simulink subsystem "drone_model"  (R2023a)
settings: Solver=VariableStepAuto  StartTime=0.0  StopTime=10.0  RelTol=1e-3
values from neighbouring files (symbols this model uses):
  G = [kF kF kF kF ... (first row only)    [config.m]
  Ginv = inv(G)    [config.m]
  k_loss = 1.219    [config.m]
  kF = -0.00019205 / 1.225    (= -0.000156775510204)    [config.m]
  kM = 4.90694039e-06 / 1.225    (= 4.00566562449e-06)    [config.m]
undefined symbols (not defined in the file or in its folder): param
libraries: shared6dof x1
settings Model: Creator=timme  LastModifiedBy=timme

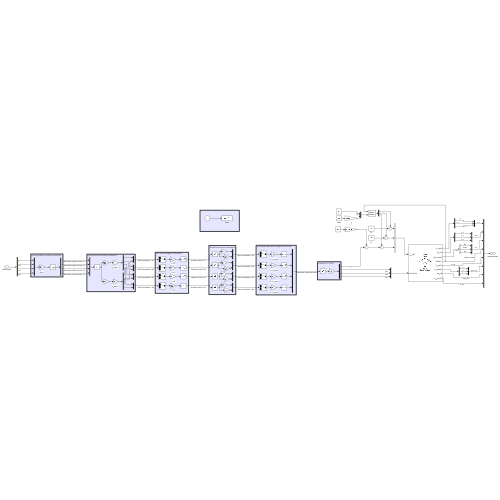
[thumbnail: Simulink's stored preview of the top-level diagram]
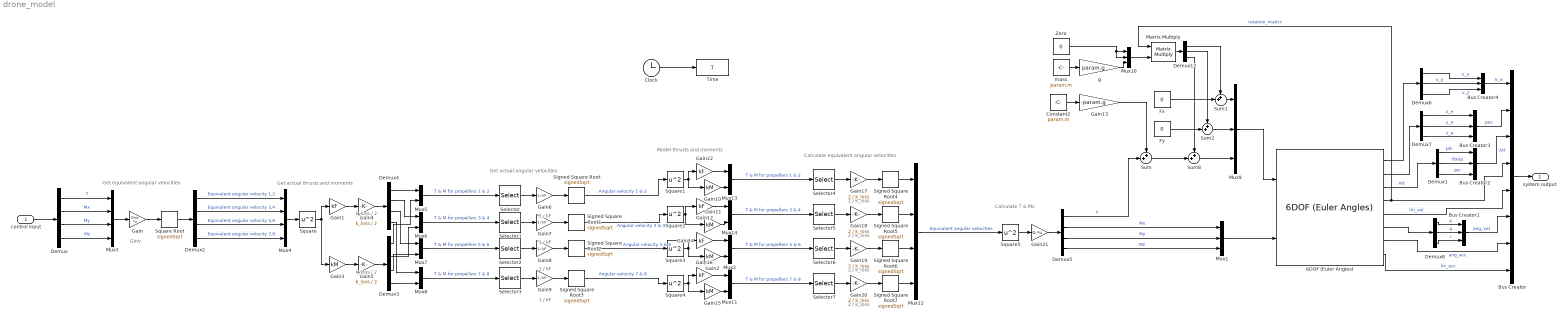
== system drone_model ==
  note: 1 / kF
  note: Calculate equivalent angular velocities
  note: Model thrusts and moments
  note: k_loss / 2
  note: Calculate T & Ms
  note: 2 / k_loss
  note: 1 / kF
  note: Get actual angular velocities
  note: Ginv
  note: Get equivalent angular velocities
  note: 1 / kF
  note: Get actual thrusts and moments
  note: 1 / kF
  note: k_loss / 2
  note: 2 / k_loss
  note: 2 / k_loss
  note: 2 / k_loss
  control input : Inport
  6DOF (Euler Angles) : shared6dof/6DOF (Euler Angles)  units=Metric (MKS)  mtype=Fixed  rep=Euler Angles  xme_0=[0 0 0]  Vm_0=[0 0 0]  eul_0=[0 0 0]  pm_0=[0 0 0]  mass_0=param.m  mass_e=0.5  mass_f=2.0  inertia=param.I  inertia_e=eye(3)  inertia_f=2*eye(3)  k_quat=1.0  vre_flag=on  abi_flag=off  aMode=0  xme_statename=''  Vm_statename=''  eul_statename=''  quat_statename=''  pm_statename=''  mass_statename=''
  Bus Creator : BusCreator  Inputs=8
  Bus Creator{1..4} (4 alike) : BusCreator  Inputs=3
  Clock : Clock
  Constant2 : Constant  Value=param.m
  Demux{,2..5} (5 alike) : Demux
  Demux{1,6..8,12} (5 alike) : Demux  Outputs=3
  Fx : Constant  Value=0
  Fy : Constant  Value=0
  Gain : Gain  Gain=Ginv  Multiplication=Matrix(K*u)
  Gain{1,12,14,16,22} (5 alike) : Gain  Gain=kF
  Gain{2..3,10..11,15} (5 alike) : Gain  Gain=kM
  Gain13 : Gain  Gain=-param.g
  Gain{17..20} (4 alike) : Gain  Gain=2 / k_loss
  Gain21 : Gain  Gain=G  Multiplication=Matrix(K*u)
  Gain4 : Gain  Gain=k_loss / 2
  Gain5 : Gain  Gain=k_loss / 2
  Gain{6..9} (4 alike) : Gain  Gain=1 / kF
  Matrix Multiply : Product  Inputs=**  Multiplication=Matrix(*)
  Mux1 : Mux  Inputs=3
  Mux10 : Mux  Inputs=3
  Mux{2,5..8,11,13..14} (8 alike) : Mux  Inputs=2
  Mux12 : Mux
  Mux3 : Mux
  Mux4 : Mux
  Mux9 : Mux  Inputs=3
  Selector{,1..7} (8 alike) : Selector  InputPortWidth=2  IndexOptions=Index vector (dialog)  Indices=1  OutputSizes=1
  Signed Square Root{,1..7} (8 alike) : Sqrt  Operator=signedSqrt
  Square : Math  Operator=square  SignedPower=on  RndMeth=Zero
  Square Root : Sqrt  Operator=signedSqrt
  Square{1..5} (5 alike) : Math  Operator=square
  Sum{,1..2,8} (4 alike) : Sum  Inputs=++|
  Time : ToWorkspace  VariableName=T  SampleTime=-1
      settings: Decimation=100
  Zero : Constant  Value=0  OutDataTypeStr=Inherit: Inherit via back propagation
  g : Gain  Gain=param.g
  mass : Constant  Value=param.m
  system output : Outport
  wires:
  Clock/1 -> Time/1
  6DOF (Euler Angles)/2 -> Demux7/1
  6DOF (Euler Angles)/8 -> Bus Creator/8  "lin_acc"
  Mux1/1 -> 6DOF (Euler Angles)/2
  6DOF (Euler Angles)/7 -> Bus Creator/7  "ang_acc"
  6DOF (Euler Angles)/4 -> Bus Creator/4, Matrix Multiply/1  "rotation_matrix"
  6DOF (Euler Angles)/1 -> Demux6/1
  6DOF (Euler Angles)/5 -> Bus Creator/5  "lin_vel"
  6DOF (Euler Angles)/6 -> Demux8/1
  6DOF (Euler Angles)/3 -> Demux1/1  "Att"
  Bus Creator/1 -> system output/1
  Demux8/3 -> Bus Creator1/3  "r"
  Demux8/2 -> Bus Creator1/2  "q"
  Demux8/1 -> Bus Creator1/1  "p"
  Demux1/3 -> Bus Creator2/3  "psi"
  Demux1/2 -> Bus Creator2/2  "theta"
  Demux1/1 -> Bus Creator2/1  "phi"
  Demux7/3 -> Bus Creator3/3  "z_e"
  Demux7/2 -> Bus Creator3/2  "y_e"
  Demux7/1 -> Bus Creator3/1  "x_e"
  Demux6/3 -> Bus Creator4/3  "v_z"
  Demux6/2 -> Bus Creator4/2  "v_y"
  Demux6/1 -> Bus Creator4/1  "v_x"
  Bus Creator4/1 -> Bus Creator/1  "V_e"
  Bus Creator1/1 -> Bus Creator/6  "ang_vel"
  Bus Creator2/1 -> Bus Creator/3  "Att"
  Bus Creator3/1 -> Bus Creator/2  "pos"
  Sum/1 -> Sum8/2
  Constant2/1 -> Gain13/1
  g/1 -> Mux10/3
  Mux10/1 -> Matrix Multiply/2
  Fx/1 -> Sum1/2
  Demux12/3 -> Sum8/1
  Demux12/2 -> Sum2/1
  Gain13/1 -> Sum/1
  Sum2/1 -> Mux9/2
  Mux9/1 -> 6DOF (Euler Angles)/1
  mass/1 -> g/1
  Demux12/1 -> Sum1/1
  Zero/1 -> Mux10/2, Mux10/1
  Sum1/1 -> Mux9/1
  Sum8/1 -> Mux9/3
  Matrix Multiply/1 -> Demux12/1
  Fy/1 -> Sum2/2
  Demux/4 -> Mux3/4  "Mz"
  control input/1 -> Demux/1
  Demux/1 -> Mux3/1  "T"
  Demux/2 -> Mux3/2  "Mx"
  Demux5/2 -> Mux1/1  "Mx"
  Demux4/1 -> Mux5/1
  Mux14/1 -> Selector5/1  "T & M for propellers 3 & 4"
  Mux12/1 -> Square5/1  "Equivalent angular velocities"
  Gain/1 -> Square Root/1
  Mux5/1 -> Selector/1  "T & M for propellers 1 & 2"
  Gain18/1 -> Signed Square Root5/1
  Selector7/1 -> Gain20/1
  Gain1/1 -> Gain4/1
  Demux/3 -> Mux3/3  "My"
  Gain21/1 -> Demux5/1
  Square5/1 -> Gain21/1
  Signed Square Root6/1 -> Mux12/3
  Gain9/1 -> Signed Square Root3/1
  Gain20/1 -> Signed Square Root7/1
  Signed Square Root5/1 -> Mux12/2
  Selector5/1 -> Gain18/1
  Demux5/3 -> Mux1/2  "My"
  Gain7/1 -> Signed Square Root1/1
  Gain19/1 -> Signed Square Root6/1
  Signed Square Root4/1 -> Mux12/1
  Gain15/1 -> Mux11/2
  Demux5/1 -> Sum/2  "T"
  Square1/1 -> Gain10/1, Gain22/1
  Demux3/3 -> Mux7/2
  Gain12/1 -> Mux14/1
  Gain22/1 -> Mux13/1
  Mux8/1 -> Selector3/1  "T & M for propellers 7 & 8"
  Gain16/1 -> Mux11/1
  Selector6/1 -> Gain19/1
  Gain14/1 -> Mux2/1
  Square2/1 -> Gain11/1, Gain12/1
  Selector4/1 -> Gain17/1
  Gain10/1 -> Mux13/2
  Selector2/1 -> Gain8/1
  Gain2/1 -> Mux2/2
  Gain8/1 -> Signed Square Root2/1
  Square3/1 -> Gain2/1, Gain14/1
  Signed Square Root3/1 -> Square4/1  "Angular velocity 7 & 8"
  Signed Square Root2/1 -> Square3/1  "Angular velocity 5 & 6"
  Demux3/4 -> Mux8/2
  Signed Square Root1/1 -> Square2/1  "Angular velocity 3 & 4"
  Signed Square Root/1 -> Square1/1  "Angular velocity 1 & 2"
  Mux7/1 -> Selector2/1  "T & M for propellers 5 & 6"
  Mux11/1 -> Selector7/1  "T & M for propellers 7 & 8"
  Mux6/1 -> Selector1/1  "T & M for propellers 3 & 4"
  Demux4/4 -> Mux8/1
  Demux4/3 -> Mux7/1
  Demux3/2 -> Mux6/2
  Demux2/3 -> Mux4/3  "Equivalent angular velocity 5,6"
  Gain11/1 -> Mux14/2
  Gain6/1 -> Signed Square Root/1
  Selector1/1 -> Gain7/1
  Demux2/2 -> Mux4/2  "Equivalent angular velocity 3,4"
  Mux13/1 -> Selector4/1  "T & M for propellers 1 & 2"
  Gain17/1 -> Signed Square Root4/1
  Square Root/1 -> Demux2/1
  Demux3/1 -> Mux5/2
  Square/1 -> Gain3/1, Gain1/1
  Selector/1 -> Gain6/1
  Mux4/1 -> Square/1
  Demux2/1 -> Mux4/1  "Equivalent angular velocity 1,2"
  Gain4/1 -> Demux4/1
  Mux2/1 -> Selector6/1  "T & M for propellers 5 & 6"
  Gain5/1 -> Demux3/1
  Demux2/4 -> Mux4/4  "Equivalent angular velocity 7,8"
  Demux4/2 -> Mux6/1
  Mux3/1 -> Gain/1
  Demux5/4 -> Mux1/3  "Mz"
  Gain3/1 -> Gain5/1
  Square4/1 -> Gain15/1, Gain16/1
  Signed Square Root7/1 -> Mux12/4
  Selector3/1 -> Gain9/1
